simulink model "Inverter (2)"  (R2024a)
settings: Solver=VariableStepAuto  StartTime=0.0  StopTime=10.0  RelTol=1e-3
libraries: slpidlib x4, spsSeriesRLCBranchLib x3, spsThreePhaseSeriesRLCBranchLib x3, spsabctodq0Lib x3, spsGroundLib x2, spsThreePhaseVIMeasurementLib x2, spsDCVoltageSourceLib x1, spsPWMGenerator2LevelLib x1, spsTwoLevelConverterLib x1, spsdq0toabcLib x1, sps_lib x1
settings Model: Creator=Mahendra  LastModifiedBy=Mahendra

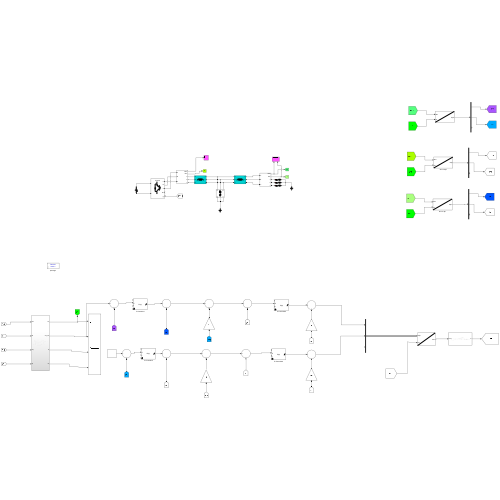
[thumbnail: Simulink's stored preview of the top-level diagram]
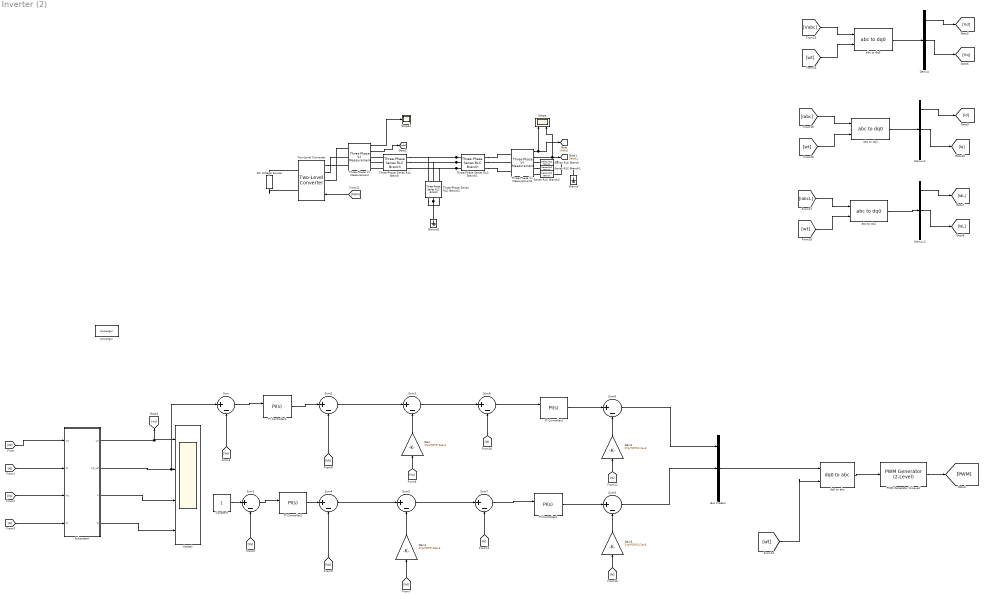
== system Inverter (2) ==
  Bus Creator : BusCreator  Inputs=3
  Constant : Constant
  DC Voltage Source : spsDCVoltageSourceLib/DC Voltage Source  Amplitude=800  Measurements=None
  Demux : Demux  Outputs=3
  Demux1 : Demux  Outputs=3
  Demux2 : Demux  Outputs=3
  Gain : Gain  Gain=2*pi*50*9.94e-6
  Gain1 : Gain  Gain=2*pi*50*9.94e-6
  Gain2 : Gain  Gain=2*pi*50*10.2e-6
  Gain3 : Gain  Gain=2*pi*50*10.2e-6
  Ground : spsGroundLib/Ground  LConnTagsString=a
  Ground1 : spsGroundLib/Ground  LConnTagsString=a
  PI Controller{1..4} (4 alike) : slpidlib/PID Controller  Controller=PI  Form=Parallel  TimeDomain=Continuous-time  UseExternalTs=off  SampleTime=-1  IntegratorMethod=Forward Euler  FilterMethod=Forward Euler  ControllerParametersSource=external  P=1  I=1  UseKiTs=off  D=0  UseExternalDerivativeSource=off  N=100  UseFilter=on  TunerSelectOption=Transfer Function Based (PID Tuner App)  InitialConditionSource=internal  InitialConditionForIntegrator=0  InitialConditionForFilter=0  DifferentiatorICPrevScaledInput=0  ExternalReset=level  TrackingMode=off  Kt=1  LimitOutput=on  SatLimitsSource=internal  UpperSaturationLimit=1  LowerSaturationLimit=-1  LinearizeAsGain=on  AntiWindupMode=clamping  Kb=1  LimitIntegrator=off  UpperIntegratorSaturationLimit=inf  LowerIntegratorSaturationLimit=-inf  RndMeth=Simplest  POutMin=[]  POutMax=[]  IOutMin=[]  IOutMax=[]  DOutMin=[]  DOutMax=[]  NOutMin=[]  NOutMax=[]  SumOutMin=[]  SumOutMax=[]  SaturationOutDataTypeStr=Inherit: Inherit via back propagation  SaturationOutMin=[]  SaturationOutMax=[]  PParamMin=[]  PParamMax=[]  IParamMin=[]  IParamMax=[]  DParamMin=[]  DParamMax=[]  NParamMin=[]  NParamMax=[]  KbParamMin=[]  KbParamMax=[]  KtParamMin=[]  KtParamMax=[]  KbOutMin=[]  KbOutMax=[]  KtOutMin=[]  KtOutMax=[]  IntegratorOutMin=[]  IntegratorOutMax=[]  FilterOutMin=[]  FilterOutMax=[]  SumI1OutMin=[]  SumI1OutMax=[]  SumI2OutMin=[]  SumI2OutMax=[]  SumI3OutMin=[]  SumI3OutMax=[]  SumI4OutMin=[]  SumI4OutMax=[]  SumDOutMin=[]  SumDOutMax=[]  DifferentiatorOutMin=[]  DifferentiatorOutMax=[]  FilterDiffOutCoefMin=[]  FilterDiffOutCoefMax=[]  ReciprocalOutMin=[]  ReciprocalOutMax=[]  SumDenOutMin=[]  SumDenOutMax=[]  SumNumOutMin=[]  SumNumOutMax=[]  DivideOutMin=[]  DivideOutMax=[]  UdiffTsProdOutMin=[]  UdiffTsProdOutMax=[]  NTsProdOutMin=[]  NTsProdOutMax=[]  UintegralTsProdOutMin=[]  UintegralTsProdOutMax=[]  UngainTsProdOutMin=[]  UngainTsProdOutMax=[]  ClampingZeroOutDataTypeStr=Inherit: Inherit via back propagation  ClampingZeroOutMin=[]  ClampingZeroOutMax=[]  FilterDenConstantOutDataTypeStr=Inherit: Inherit via back propagation  FilterDenConstantOutMin=[]  FilterDenConstantOutMax=[]  PCopyOutDataTypeStr=Inherit: Inherit via back propagation  PCopyOutMin=[]  PCopyOutMax=[]  NCopyOutDataTypeStr=Inherit: Inherit via back propagation  NCopyOutMin=[]  NCopyOutMax=[]  IntegratorContinuousStateAttributes=''  IntegratorStateMustResolveToSignalObject=off  IntegratorRTWStateStorageClass=Auto  FilterContinuousStateAttributes=''  FilterStateMustResolveToSignalObject=off  FilterRTWStateStorageClass=Auto  ParallelPVariant=ExternalParameters  IdealPVariant=Disabled  IVariant=ExternalParameters  DVariant=Disabled  IntegratorVariant=Continuous  SatVariant=Enabled  AWVariant=ContClampingParallel  PCopyVariant=Disabled  TRVariant=Disabled  FdbkBlocksVariant=Forward  IdealPFdbkVariant=Disabled  SatFdbkVariant=Disabled  DerivativeFilterVariant=Disabled  NVariant=Disabled  NCopyVariant=Disabled_SignalSpec  FilterICVariant=Disabled  IntegratorICVariant=InternalICs  ExternalResetVariant=ExternalReset  TRSumVariant=Passthrough  SumFdbkVariant=Disabled  SumVariant=Sum_PI  TsampFilterVariant=InternalTs  TsampNgainVariant=Passthrough  TsampIntegralVariant=Disabled_SignalSpec  ExternalSaturationOutDataTypeStr=Inherit: Same as second input  DerivativeSourceVariant=Disabled
      settings: LibrarySourceBlock=mcbhdllib/Controls/Controllers/PI Controller
  PWM Generator (2-Level) : spsPWMGenerator2LevelLib/PWM Generator (2-Level)  ModulatorType=Three-phase bridge (6 pulses)  ModulatorMode=Unsynchronized  Fc=27*50  Pc=90  nF=27  MinMax="[ -1  1 ]"  SamplingTechnique=Natural  ModulatingSignals=off  m=0.8  Freq=60  Phase=0  Ts=0  ShowCarrierOutport=off
  Scope : Scope  NumInputPorts=2
  Scope1 : Scope
  Scope2 : Scope  NumInputPorts=4
  Series RLC Branch : spsSeriesRLCBranchLib/Series RLC Branch  LConnTagsString=__new0  RConnTagsString=__new0  BranchType=RL  Resistance=100  Inductance=10e-3  SetiL0=off  InitialCurrent=0  Capacitance=1e-6  Setx0=off  InitialVoltage=0  Measurements=None
  Series RLC Branch1 : spsSeriesRLCBranchLib/Series RLC Branch  LConnTagsString=__new0  RConnTagsString=__new0  BranchType=RL  Resistance=100  Inductance=10e-3  SetiL0=off  InitialCurrent=0  Capacitance=1e-6  Setx0=off  InitialVoltage=0  Measurements=None
  Series RLC Branch2 : spsSeriesRLCBranchLib/Series RLC Branch  LConnTagsString=__new0  RConnTagsString=__new0  BranchType=RL  Resistance=100  Inductance=10e-3  SetiL0=off  InitialCurrent=0  Capacitance=1e-6  Setx0=off  InitialVoltage=0  Measurements=None
  Subsystem : Subsystem
  Sum{,1..9} (10 alike) : Sum  Inputs=|+-
  Three-Phase Series RLC Branch : spsThreePhaseSeriesRLCBranchLib/Three-Phase Series RLC Branch  LConnTagsString=A|B|C  RConnTagsString=A|B|C  BranchType=L  Resistance=1  Inductance=5.1e-3  Capacitance=1e-6  Measurements=None
  Three-Phase Series RLC Branch1 : spsThreePhaseSeriesRLCBranchLib/Three-Phase Series RLC Branch  LConnTagsString=A|B|C  RConnTagsString=A|B|C  BranchType=L  Resistance=1  Inductance=5.1e-3  Capacitance=1e-6  Measurements=None
  Three-Phase Series RLC Branch2 : spsThreePhaseSeriesRLCBranchLib/Three-Phase Series RLC Branch  LConnTagsString=A|B|C  RConnTagsString=A|B|C  BranchType=RC  Resistance=5.37  Inductance=5.1e-3  Capacitance=9.94e-6  Measurements=None
  Three-Phase V-I Measurement : spsThreePhaseVIMeasurementLib/Three-Phase V-I Measurement  VoltageMeasurement=phase-to-phase  SetLabelV=off  LabelV=Vabc  Vpu=off  VpuLL=off  CurrentMeasurement=yes  SetLabelI=off  LabelI=Iabc  Ipu=off  Pbase=100e6  Vbase=500e3  OutputType=Complex  PhasorSimulation=off  PSBequivalent=0
  Three-Phase V-I Measurement1 : spsThreePhaseVIMeasurementLib/Three-Phase V-I Measurement  VoltageMeasurement=phase-to-phase  SetLabelV=off  LabelV=Vabc  Vpu=off  VpuLL=off  CurrentMeasurement=yes  SetLabelI=off  LabelI=Iabc  Ipu=off  Pbase=100e6  Vbase=500e3  OutputType=Complex  PhasorSimulation=off  PSBequivalent=0
  Two-Level Converter : spsTwoLevelConverterLib/Two-Level Converter  ModelType=Switching devices  Ron=1e-3  Rs=1e6  Cs=inf  Vforward=[0,0]  Ron_Diode=1e-3  Rs_Diode=1e6  Cs_Diode=inf  Vf_Diode=1e-3  Rs_CurrentSource=inf  Ron_ACsource=1e-3
      settings: LibrarySourceBlock=sps_lib/Power Electronics/Two-Level Converter
  abc to dq0 : spsabctodq0Lib/abc to dq0  Alignment=90 degrees behind phase A axis
  abc to dq1 : spsabctodq0Lib/abc to dq0  Alignment=90 degrees behind phase A axis
  abc to dq2 : spsabctodq0Lib/abc to dq0  Alignment=90 degrees behind phase A axis
  dq0 to abc : spsdq0toabcLib/dq0 to abc  Alignment=90 degrees behind phase A axis
  powergui : sps_lib/powergui  Priority=1  SimulationMode=Discrete  SampleTime=1e-6  frequency=60  Iterations=50  frequencyindice=0  Pbase=100e6  ErrMax=1e-4  UnitsV=kV  UnitsW=MW  buscounter=0  FunctionMessages=off  echomessages=off  EnableUseOfTLC=off  CurrentSourceSwitches=off  DisableSnubberDevices=off  DisableRonSwitches=off  DisableVfSwitches=off  DisplayEquations=off  AutomaticDiscreteSolvers=off  SolverType=Tustin/Backward Euler (TBE)  Interpol=off  ExternalGateDelay=off  methode=off  Ts=100  x0status=blocks  SPID=on  SwTol=0  HookPort=off  NonlinearTolerance=1e-4  nMaxIteration=100  ContinueOnMaxIteration=off  RestoreLinks=warning  ResistiveCurrentMeasurement=off  Frange=[0:2:500]  Ylog=off  Xlog=on  ShowGrid=off  save=off  variable=ZData  structure=0  ZoomFFT=off  StartTime=0.0  cycles=1  DisplayStyle=1  fundamental=60  FreqAxis=off  MaxFrequency=1000  frequencyindicesteady=1  RmsSteady=1  display=off
  wires:
  Demux/2 -> [Vq]
  [wt] -> abc to dq0/2
  Demux2/2 -> [IqL]
  Demux2/1 -> [IdL]
  abc to dq1/1 -> Demux2/1
  [IabcL] -> abc to dq1/1
  [wt] -> abc to dq1/2
  dq0 to abc/1 -> PWM Generator (2-Level)/1
  [Id] -> Gain3/1
  Gain3/1 -> Sum9/2
  [IqL] -> Sum4/2
  [IdL] -> Sum2/2
  Gain/1 -> Sum3/2
  Sum4/1 -> Sum5/1
  Subsystem/4(Q) -> Scope2/4
  Subsystem/2(Vd_ref) -> Sum/1, Scope2/2
  Subsystem/1(wt) -> [wt], Scope2/1
  Demux1/1 -> [Id]
  [wt] -> abc to dq2/2
  abc to dq2/1 -> Demux1/1
  Sum5/1 -> Sum7/1
  Sum3/1 -> Sum6/1
  [Vd] -> Subsystem/1(Vd)
  [Id] -> Subsystem/2(Id)
  [Vd] -> Gain1/1
  [Vabc] -> abc to dq0/1
  [Iq] -> Sum7/2
  [Id] -> Sum6/2
  [Vq] -> Subsystem/3(Vq)
  [Vq] -> Gain/1
  Gain2/1 -> Sum8/2
  abc to dq0/1 -> Demux/1
  [Vq] -> Sum1/2
  Demux1/2 -> [Iq]
  Gain1/1 -> Sum5/2
  Subsystem/3(P) -> Scope2/3
  Sum9/1 -> Bus Creator/2
  Sum8/1 -> Bus Creator/1
  [Iq] -> Gain2/1
  [Iabc] -> abc to dq2/1
  Bus Creator/1 -> dq0 to abc/1
  Three-Phase V-I Measurement/2 -> [Iabc]
  Three-Phase V-I Measurement1/2 -> Scope/2, [IabcL]
  Three-Phase V-I Measurement/1 -> Scope1/1
  Demux/1 -> [Vd]
  [Vd] -> Sum/2
  Three-Phase V-I Measurement1/1 -> [Vabc], Scope/1
  [Iq] -> Subsystem/4(Iq)
  PWM Generator (2-Level)/1 -> [PWM]
  [wt] -> dq0 to abc/2
  Constant/1 -> Sum1/1
  Sum2/1 -> Sum3/1
  PI Controller1/1 -> Sum2/1
  Sum/1 -> PI Controller1/2
  Sum1/1 -> PI Controller2/2
  PI Controller2/1 -> Sum4/1
  Sum6/1 -> PI Controller3/2
  PI Controller3/1 -> Sum8/1
  Sum7/1 -> PI Controller4/2
  PI Controller4/1 -> Sum9/1
  [PWM] -> Two-Level Converter/1
  connections:
  Three-Phase Series RLC Branch2/RConn2 -- Three-Phase Series RLC Branch2/RConn1 -- Ground1/LConn1 -- Three-Phase Series RLC Branch2/RConn3
  Three-Phase Series RLC Branch1/LConn2 -- Three-Phase Series RLC Branch/RConn2 -- Three-Phase Series RLC Branch2/LConn2
  Series RLC Branch/RConn1 -- Series RLC Branch1/RConn1 -- Ground/LConn1 -- Series RLC Branch2/RConn1
  Three-Phase Series RLC Branch1/LConn1 -- Three-Phase Series RLC Branch/RConn1 -- Three-Phase Series RLC Branch2/LConn1
  Three-Phase Series RLC Branch1/LConn3 -- Three-Phase Series RLC Branch/RConn3 -- Three-Phase Series RLC Branch2/LConn3
  Two-Level Converter/LConn1 -- Three-Phase V-I Measurement/LConn1
  Three-Phase Series RLC Branch1/RConn1 -- Three-Phase V-I Measurement1/LConn1
  Three-Phase V-I Measurement1/RConn3 -- Series RLC Branch2/LConn1
  Three-Phase Series RLC Branch1/RConn2 -- Three-Phase V-I Measurement1/LConn2
  Three-Phase Series RLC Branch1/RConn3 -- Three-Phase V-I Measurement1/LConn3
  Three-Phase V-I Measurement1/RConn1 -- Series RLC Branch/LConn1
  Three-Phase V-I Measurement1/RConn2 -- Series RLC Branch1/LConn1
  Three-Phase Series RLC Branch/LConn2 -- Three-Phase V-I Measurement/RConn2
  Three-Phase Series RLC Branch/LConn1 -- Three-Phase V-I Measurement/RConn1
  Two-Level Converter/LConn2 -- Three-Phase V-I Measurement/LConn2
  Two-Level Converter/LConn3 -- Three-Phase V-I Measurement/LConn3
  DC Voltage Source/RConn1 -- Two-Level Converter/RConn1
  DC Voltage Source/LConn1 -- Two-Level Converter/RConn2
  Three-Phase Series RLC Branch/LConn3 -- Three-Phase V-I Measurement/RConn3

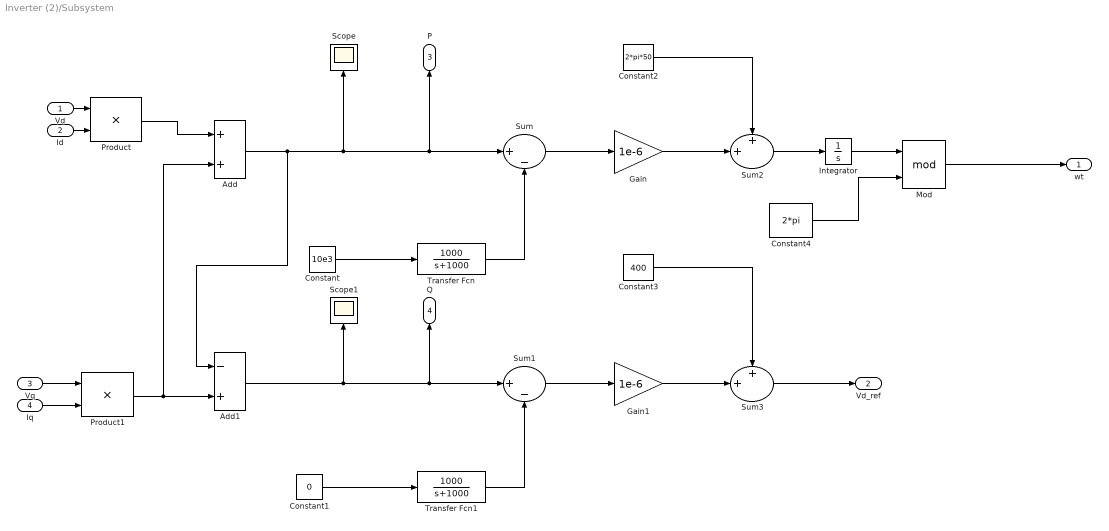
== system Inverter (2)/Subsystem ==
  Vd : Inport
  Id : Inport  Port=2
  Vq : Inport  Port=3
  Iq : Inport  Port=4
  Add : Sum
  Add1 : Sum  Inputs=-+
  Constant : Constant  Value=10e3
  Constant1 : Constant  Value=0
  Constant2 : Constant  Value=2*pi*50
  Constant3 : Constant  Value=400
  Constant4 : Constant  Value=2*pi
  Gain : Gain  Gain=1e-6
  Gain1 : Gain  Gain=1e-6
  Integrator : Integrator
  Mod : Math  Operator=mod
  Product : Product
  Product1 : Product
  Scope : Scope
  Scope1 : Scope
  Sum : Sum  Inputs=|+-
  Sum1 : Sum  Inputs=|+-
  Sum2 : Sum  Inputs=++|
  Sum3 : Sum  Inputs=++|
  Transfer Fcn : TransferFcn  Numerator=[1000]  Denominator=[1 1000]
  Transfer Fcn1 : TransferFcn  Numerator=[1000]  Denominator=[1 1000]
  wt : Outport
  Vd_ref : Outport  Port=2
  P : Outport  Port=3
  Q : Outport  Port=4
  wires:
  Vd/1 -> Product/1
  Id/1 -> Product/2
  Iq/1 -> Product1/2
  Vq/1 -> Product1/1
  Product1/1 -> Add1/2, Add/2
  Constant/1 -> Transfer Fcn/1
  Constant1/1 -> Transfer Fcn1/1
  Product/1 -> Add/1
  Transfer Fcn/1 -> Sum/2
  Transfer Fcn1/1 -> Sum1/2
  Add1/1 -> Scope1/1, Q/1, Sum1/1
  Add/1 -> Add1/1, Scope/1, P/1, Sum/1
  Sum/1 -> Gain/1
  Sum1/1 -> Gain1/1
  Gain1/1 -> Sum3/2
  Gain/1 -> Sum2/2
  Constant2/1 -> Sum2/1
  Constant3/1 -> Sum3/1
  Sum2/1 -> Integrator/1
  Integrator/1 -> Mod/1
  Mod/1 -> wt/1
  Constant4/1 -> Mod/2
  Sum3/1 -> Vd_ref/1
